simulink model "simulink_1_manoel"  (R2018a)
settings: Solver=VariableStepAuto  StartTime=0.0  StopTime=10.0  RelTol=1e-3
libraries: simulink x1
settings Model: Creator=joaovitor  LastModifiedBy=joaovitor

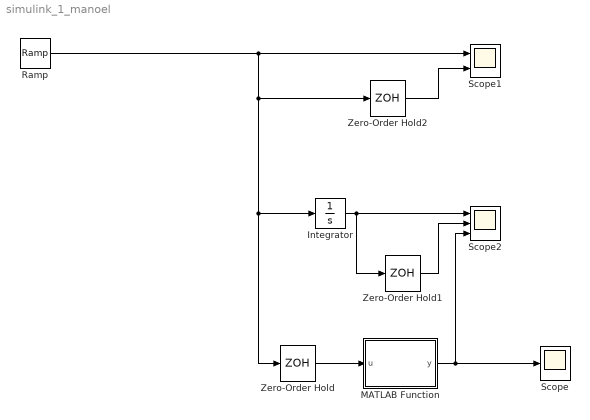
== system simulink_1_manoel ==
  Integrator : Integrator
  MATLAB Function : MATLAB Function  TreatAsAtomicUnit=on
  Ramp : simulink/Sources/Ramp  slope=1  start=0  InitialOutput=0
  Scope : Scope
  Scope1 : Scope  NumInputPorts=2
  Scope2 : Scope  NumInputPorts=3
  Zero-Order Hold : ZeroOrderHold  SampleTime=-1
  Zero-Order Hold1 : ZeroOrderHold  SampleTime=-1
  Zero-Order Hold2 : ZeroOrderHold  SampleTime=-1
  wires:
  Ramp/1 -> Zero-Order Hold2/1, Zero-Order Hold/1, Integrator/1, Scope1/1
  Integrator/1 -> Zero-Order Hold1/1, Scope2/1
  MATLAB Function/1(y) -> Scope2/3, Scope/1
  Zero-Order Hold2/1 -> Scope1/2
  Zero-Order Hold1/1 -> Scope2/2
  Zero-Order Hold/1 -> MATLAB Function/1(u)

== matlab function simulink_1_manoel/MATLAB Function ==
  data: u input; y output
function y = fcn(u)

y = u;
